simulink model "harmonic"  (R2018b)
settings: Solver=VariableStepAuto  StartTime=0.0  StopTime=3.6  RelTol=1e-3
libraries: simulink_extras x1
settings Model: Creator=Ali  LastModifiedBy=Ali

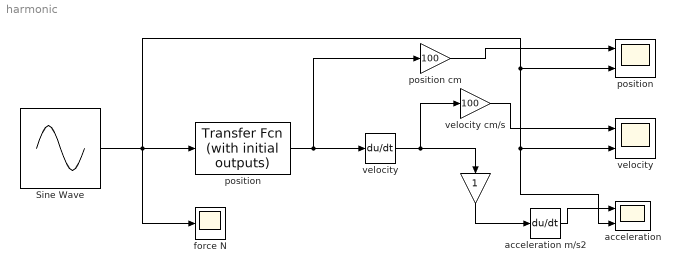
== system harmonic ==
  " " : Gain
  Sine Wave : Sin  Amplitude=20  Frequency=5  SampleTime=0
  "acceleration " : Scope  NumInputPorts=2
  acceleration m/s2 : Derivative
  "force N " : Scope
  position : simulink_extras/Additional Linear/Transfer Fcn (with initial outputs)  N=[1]  D=[1 10 100]  Y0=0  U0=0
  "position " : Scope  NumInputPorts=2
  position cm : Gain  Gain=100
  velocity : Derivative
  "velocity " : Scope  NumInputPorts=2
  velocity cm/s : Gain  Gain=100
  wires:
  position cm/1 -> "position "/1
  velocity/1 -> velocity cm/s/1, " "/1
  velocity cm/s/1 -> "velocity "/1
  position/1 -> position cm/1, velocity/1
  Sine Wave/1 -> "acceleration "/2, "velocity "/2, "position "/2, position/1, "force N "/1
  acceleration m/s2/1 -> "acceleration "/1
  " "/1 -> acceleration m/s2/1
